simulink library "rsa"  (Simulink 8.1)
settings: Solver=ode1  StartTime=0.0  StopTime=Inf  FixedStep=0.001  RelTol=1e-3
PostLoadFcn:
  | , if any(exist('dsrtsu_mdlpostloadfcn', 'file') == [2, 3, 6]), try dsrtsu_mdlpostloadfcn('Execute', bdroot); catch fprintf('Error in PostLoadFcn (dsrtsu_mdlpostloadfcn) for model "%s":\n %s\n', bdroot, lasterr); end, end,
undefined symbols (not defined in the file or in its folder): C_TICK_TIME_S, KACC_ACCRefSpdLongInt_s, KACC_ACCRefSpdRollAvgMargin_kph, KACC_ACCRefSpdShortInt_s, KACC_ACCRefSpdTimer_s, TRUE, ZERO_INT
libraries: hcu_lib x2
settings Model: DSRTSU_INTERNAL_RTI_VER=450  DSRTSU_INTERNAL_RTI_TYPE=rti1401  RTICANMMDATA=struct('GeneralSetupData',struct('modelroot','D:\ELN150201_TAIWAN\trunk\AdasDragon\software\sw_development\arch\app\acc','generalsettings',struct('filesettings',struct('destfolder',struct('Name','RTICANMM_FILES','Check',1),'buildfolder',struct('Name','.','Check',1),'AbsDestfolder',struct('Name','D:\ELN150201_TAIWAN\trunk\AdasDragon\software\sw_development\arch\app\acc\RTICANMM_FILES'),'AbsBuildfolder',struct('Name','D:\ELN150201_TAIWAN\trunk\AdasDragon\software\sw_development\arch\app\acc'))),'options',struct('addpaths',1,'rmpaths',1,'addtrcexclusion',logical(1),'cannavigator',struct('checkmonitoring',0),'show_usrtrc',0,'use_usrtrc',0),'advanced',struct('options',[1 1 1 1 1 1 1 1 1 1 1 1 1 1 1 1 1 1 1 1 1 1 1 1 1 1 1 1 1 1 1 1 1 1 1 1 1 1 1 1 1 1 1 1 1 1 1 1 1 1 1 1 1 1 1 1 1 1 1 1 1 1 1 1 1 1 1 1 1 1 1 1 1 1 1 1 1 1 1 1 1 1 1 1 1 1 1 1 1 1 1 1 1 1 1 1 1 1 1 1]),'MPSetup',{{}},'modelname','rsa','block','rsa'))  DSRTSU_INTERNAL_RTIFPGA=40  Creator=AT015086  LastModifiedBy=AT015555

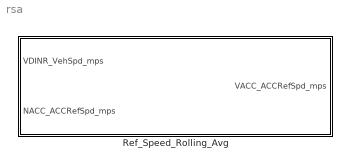
== system rsa ==
  Ref_Speed_Rolling_Avg : Subsystem

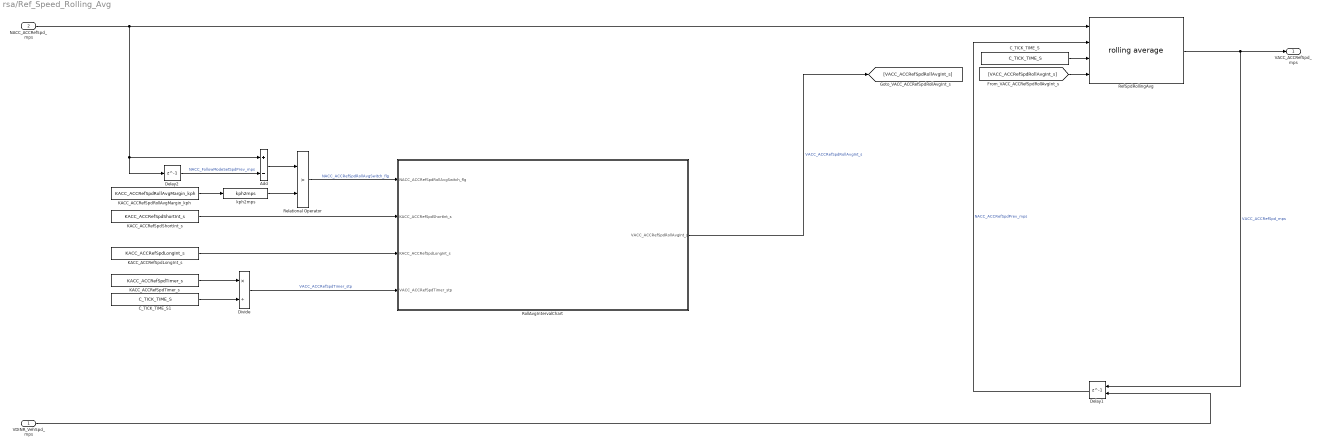
== system rsa/Ref_Speed_Rolling_Avg ==
  VDINR_VehSpd_mps : Inport
  NACC_ACCRefSpd_mps : Inport  Port=2
  Add : Sum  Inputs=+-
  C_TICK_TIME_S : Constant  Value=C_TICK_TIME_S
  C_TICK_TIME_S1 : Constant  Value=C_TICK_TIME_S
  Delay1 : Delay  DelayLength=1  InitialConditionSource=Input port
      settings: InputPortMap=u0,p4
  Delay2 : Delay  DelayLength=1
  Divide : Product  Inputs=*/
  KACC_ACCRefSpdLongInt_s : Constant  Value=KACC_ACCRefSpdLongInt_s
  KACC_ACCRefSpdRollAvgMargin_kph : Constant  Value=KACC_ACCRefSpdRollAvgMargin_kph
  KACC_ACCRefSpdShortInt_s : Constant  Value=KACC_ACCRefSpdShortInt_s
  KACC_ACCRefSpdTimer_s : Constant  Value=KACC_ACCRefSpdTimer_s
  RefSpdRollingAvg : hcu_lib/rolling average
  Relational Operator : RelationalOperator  Operator=>  OutDataTypeStr=boolean
  RollAvgIntervalChart : Stateflow chart  TreatAsAtomicUnit=on
  kph2mps : hcu_lib/kph2mps
  VACC_ACCRefSpd_mps : Outport
  wires:
  RollAvgIntervalChart/1(VACC_ACCRefSpdRollAvgInt_s) -> [VACC_ACCRefSpdRollAvgInt_s]  "VACC_ACCRefSpdRollAvgInt_s"
  Relational Operator/1 -> RollAvgIntervalChart/1(NACC_ACCRefSpdRollAvgSwitch_flg)  "NACC_ACCRefSpdRollAvgSwitch_flg"
  kph2mps/1 -> Relational Operator/2
  Add/1 -> Relational Operator/1
  KACC_ACCRefSpdRollAvgMargin_kph/1 -> kph2mps/1
  Delay2/1 -> Add/2  "NACC_FollowModeSetSpdPrev_mps"
  KACC_ACCRefSpdLongInt_s/1 -> RollAvgIntervalChart/3(KACC_ACCRefSpdLongInt_s)
  KACC_ACCRefSpdShortInt_s/1 -> RollAvgIntervalChart/2(KACC_ACCRefSpdShortInt_s)
  Divide/1 -> RollAvgIntervalChart/4(VACC_ACCRefSpdTimer_stp)  "VACC_ACCRefSpdTimer_stp"
  C_TICK_TIME_S1/1 -> Divide/2
  KACC_ACCRefSpdTimer_s/1 -> Divide/1
  Delay1/1 -> RefSpdRollingAvg/2  "NACC_ACCRefSpdPrev_mps"
  C_TICK_TIME_S/1 -> RefSpdRollingAvg/3
  NACC_ACCRefSpd_mps/1 -> Add/1, Delay2/1, RefSpdRollingAvg/1
  RefSpdRollingAvg/1 -> VACC_ACCRefSpd_mps/1, Delay1/1  "VACC_ACCRefSpd_mps"
  [VACC_ACCRefSpdRollAvgInt_s] -> RefSpdRollingAvg/4
  VDINR_VehSpd_mps/1 -> Delay1/2

== stateflow chart Ref_Speed_Rolling_Avg/RollAvgIntervalChart ==
  state SHORT_INT
    en:
    VACC_ACCRefSpdRollAvgInt_s = KACC_ACCRefSpdShortInt_s;
  state LONG_INT
    en:
    VACC_ACCRefSpdRollAvgInt_s = KACC_ACCRefSpdLongInt_s;
    NACC_ACCRollAvgTimerLocal_stp= ZERO_INT;
    du:
    NACC_ACCRollAvgTimerLocal_stp = NACC_ACCRollAvgTimerLocal_stp+1;
  (default) -> SHORT_INT
  SHORT_INT -> LONG_INT : [NACC_ACCRefSpdRollAvgSwitch_flg==TRUE]
  LONG_INT -> SHORT_INT : [NACC_ACCRollAvgTimerLocal_stp>VACC_ACCRefSpdTimer_stp]
  data: NACC_ACCRefSpdRollAvgSwitch_flg input double; KACC_ACCRefSpdShortInt_s input double; KACC_ACCRefSpdLongInt_s input double; VACC_ACCRefSpdTimer_stp input double; VACC_ACCRefSpdRollAvgInt_s output single; ZERO_INT parameter boolean; TRUE parameter boolean; NACC_ACCRollAvgTimerLocal_stp local single
